simulink model "TwoLevel_ThreePhase_PWM_2017b"  (R2017b)
settings: Solver=VariableStepAuto  StartTime=0.0  StopTime=0.1  RelTol=1e-3
StopFcn:
  | Vabc=out.Vabcn;
  | Vab=out.Vab;
  | Iabc=out.Iabcn;
libraries: powerlib x12, simulink x4
settings Model: Creator=defus  LastModifiedBy=Mehdi
settings DataIOCC: ReturnWorkspaceOutputs=on
settings DebuggingCC: UnconnectedInputMsg=none  UnconnectedOutputMsg=none  UnconnectedLineMsg=none
settings ModelReferenceCC: EnableRefExpFcnMdlSchedulingChecks=off
settings SFSimCC: SimUseLocalCustomCode=on
settings RTWCC: Description=Generic Real-Time Target  RTWUseLocalCustomCode=on
settings CodeAppCC: StateflowObjectComments=on
settings SimscapeCC: SimscapeNormalizeSystem=off

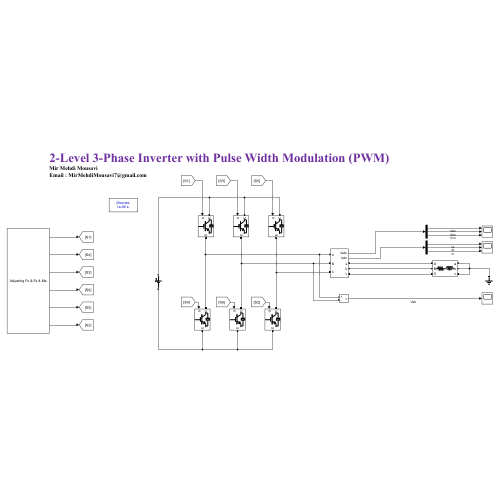
[thumbnail: Simulink's stored preview of the top-level diagram]
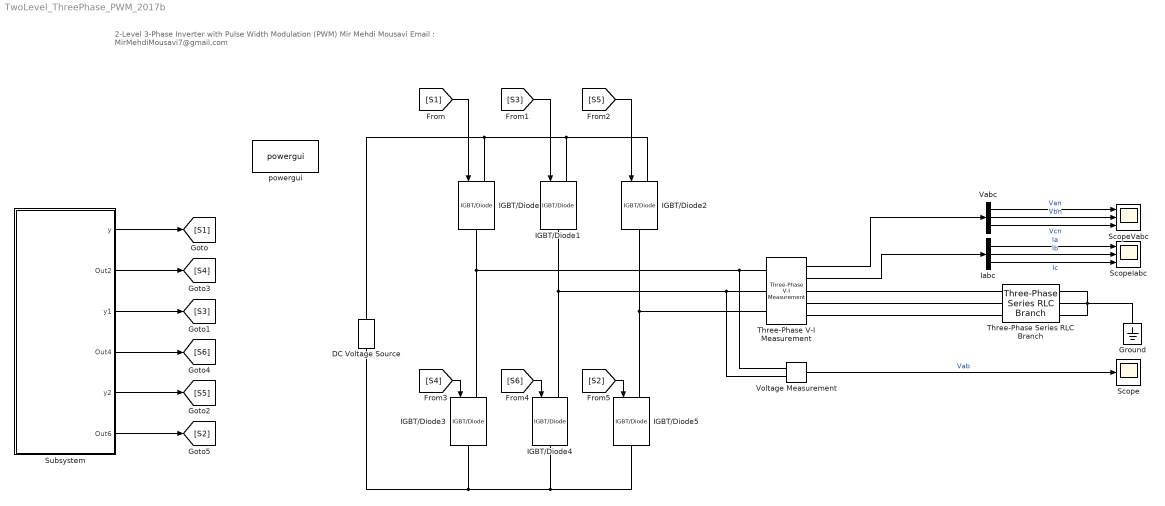
== system TwoLevel_ThreePhase_PWM_2017b ==
  note: 2-Level 3-Phase Inverter with Pulse Width Modulation (PWM)
      | Mir Mehdi Mousavi
      | Email : MirMehdiMousavi7@gmail.com
  DC Voltage Source : powerlib/Electrical Sources/DC Voltage Source  Amplitude=400  Measurements=None
  Ground : powerlib/Elements/Ground  LConnTagsString=a
  IGBT/Diode{,1..5} (6 alike) : powerlib/Power Electronics/IGBT//Diode  Ron=1e-3  Rs=1e5  Cs=inf  Measurements=off
  Iabc : Demux  Outputs=3
  Scope : Scope
  ScopeIabc : Scope  NumInputPorts=3
  ScopeVabc : Scope  NumInputPorts=3
  Subsystem : Subsystem  mask{fo=50, fs=1750, ma=1}
      mask prompts: fo "Output Frequency (Hz)"; fs "Sitching Frequency (Hz)"; ma "Index Modulation"
      mask Display: fprintf('Adjusting Fo & Fs & Ma')
  Three-Phase Series RLC Branch : powerlib/Elements/Three-Phase Series RLC Branch  LConnTagsString=A|B|C  RConnTagsString=A|B|C  BranchType=RL  Resistance=3  Inductance=1.5e-2  Capacitance=1e-6  Measurements=None
  Three-Phase V-I Measurement : powerlib/Measurements/Three-Phase V-I Measurement  VoltageMeasurement=phase-to-ground  SetLabelV=off  LabelV=Vabc  Vpu=off  VpuLL=off  CurrentMeasurement=yes  SetLabelI=off  LabelI=Iabc  Ipu=off  Pbase=100e6  Vbase=500e3  OutputType=Complex  PhasorSimulation=off  PSBequivalent=0
  Vabc : Demux  Outputs=3
  Voltage Measurement : powerlib/Measurements/Voltage Measurement  PhasorSimulation=off  OutputType=Complex  PSBequivalent=0
  powergui : powerlib/powergui  Priority=1  SimulationMode=Discrete  SampleTime=1e-6  frequency=60  Iterations=50  frequencyindice=0  Pbase=100e6  ErrMax=1e-4  UnitsV=kV  UnitsW=MW  buscounter=0  FunctionMessages=off  echomessages=off  EnableUseOfTLC=off  CurrentSourceSwitches=off  DisableSnubberDevices=off  DisableRonSwitches=off  DisableVfSwitches=off  DisplayEquations=off  AutomaticDiscreteSolvers=off  SolverType=Tustin/Backward Euler (TBE)  Interpol=off  ExternalGateDelay=off  methode=off  Ts=100  x0status=blocks  SPID=on  SwTol=0  HookPort=off  NonlinearTolerance=1e-4  nMaxIteration=100  ContinueOnMaxIteration=off  RestoreLinks=warning  ResistiveCurrentMeasurement=off  Frange=[0:2:500]  Ylog=off  Xlog=on  ShowGrid=off  save=off  variable=ZData  structure=0  ZoomFFT=off  StartTime=0.0  cycles=1  DisplayStyle=1  fundamental=60  FreqAxis=off  MaxFrequency=1000  frequencyindicesteady=1  RmsSteady=1  display=off
  wires:
  [S1] -> IGBT/Diode/1
  [S3] -> IGBT/Diode1/1
  [S5] -> IGBT/Diode2/1
  [S4] -> IGBT/Diode3/1
  [S2] -> IGBT/Diode5/1
  [S6] -> IGBT/Diode4/1
  Subsystem/1(y) -> [S1]
  Subsystem/2(Out2) -> [S4]
  Subsystem/3(y1) -> [S3]
  Subsystem/4(Out4) -> [S6]
  Subsystem/5(y2) -> [S5]
  Subsystem/6(Out6) -> [S2]
  Vabc/2 -> ScopeVabc/2  "Vbn"
  Three-Phase V-I Measurement/1 -> Vabc/1
  Three-Phase V-I Measurement/2 -> Iabc/1
  Voltage Measurement/1 -> Scope/1  "Vab"
  Iabc/2 -> ScopeIabc/2  "Ib"
  Vabc/1 -> ScopeVabc/1  "Van"
  Vabc/3 -> ScopeVabc/3  "Vcn"
  Iabc/1 -> ScopeIabc/1  "Ia"
  Iabc/3 -> ScopeIabc/3  "Ic"
  connections:
  IGBT/Diode/LConn1 -- DC Voltage Source/RConn1 -- IGBT/Diode2/LConn1 -- IGBT/Diode1/LConn1
  DC Voltage Source/LConn1 -- IGBT/Diode3/RConn1 -- IGBT/Diode5/RConn1 -- IGBT/Diode4/RConn1
  IGBT/Diode/RConn1 -- Voltage Measurement/LConn1 -- Three-Phase V-I Measurement/LConn1 -- IGBT/Diode3/LConn1
  IGBT/Diode1/RConn1 -- Voltage Measurement/LConn2 -- Three-Phase V-I Measurement/LConn2 -- IGBT/Diode4/LConn1
  IGBT/Diode2/RConn1 -- IGBT/Diode5/LConn1 -- Three-Phase V-I Measurement/LConn3
  Three-Phase Series RLC Branch/RConn3 -- Three-Phase Series RLC Branch/RConn2 -- Ground/LConn1 -- Three-Phase Series RLC Branch/RConn1
  Three-Phase V-I Measurement/RConn2 -- Three-Phase Series RLC Branch/LConn2
  Three-Phase V-I Measurement/RConn1 -- Three-Phase Series RLC Branch/LConn1
  Three-Phase V-I Measurement/RConn3 -- Three-Phase Series RLC Branch/LConn3

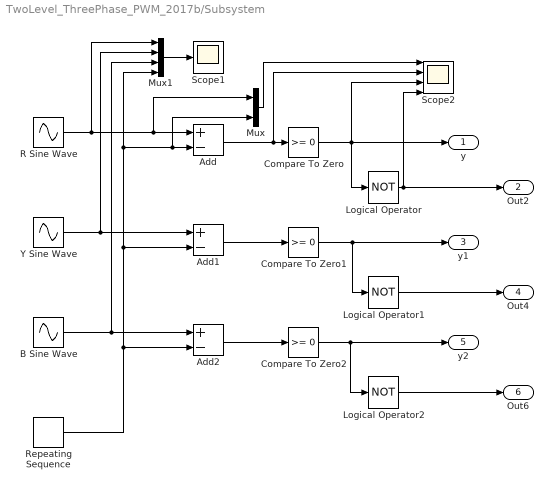
== system TwoLevel_ThreePhase_PWM_2017b/Subsystem ==
  Add : Sum  Inputs=+-
  Add1 : Sum  Inputs=+-
  Add2 : Sum  Inputs=+-
  B Sine Wave : Sin  Amplitude=ma  Frequency=2*pi*fo  Phase=-2*pi/3  SampleTime=1e-06
  Compare To Zero : simulink/Logic and Bit Operations/Compare To Zero  relop=>=  OutDataTypeStr=boolean
  Compare To Zero1 : simulink/Logic and Bit Operations/Compare To Zero  relop=>=  OutDataTypeStr=boolean
  Compare To Zero2 : simulink/Logic and Bit Operations/Compare To Zero  relop=>=  OutDataTypeStr=boolean
  Logical Operator : Logic  Operator=NOT  AllPortsSameDT=off  OutDataTypeStr=boolean
  Logical Operator1 : Logic  Operator=NOT  AllPortsSameDT=off  OutDataTypeStr=boolean
  Logical Operator2 : Logic  Operator=NOT  AllPortsSameDT=off  OutDataTypeStr=boolean
  Mux : Mux  Inputs=2
  Mux1 : Mux
  R Sine Wave : Sin  Amplitude=ma  Frequency=2*pi*fo  SampleTime=1e-06
  Repeating Sequence : simulink/Sources/Repeating Sequence  rep_seq_t=[0 1 2 3 4]*[1/(4*fs)]  rep_seq_y=[0 1 0 -1 0]
  Scope1 : Scope
  Scope2 : Scope  NumInputPorts=4
  Y Sine Wave : Sin  Amplitude=ma  Frequency=2*pi*fo  Phase=2*pi/3  SampleTime=1e-06
  y : Outport
  Out2 : Outport  Port=2
  y1 : Outport  Port=3
  Out4 : Outport  Port=4
  y2 : Outport  Port=5
  Out6 : Outport  Port=6
  wires:
  Add2/1 -> Compare To Zero2/1
  Repeating Sequence/1 -> Mux1/4, Mux/2, Add/2, Add1/2, Add2/2
  Add1/1 -> Compare To Zero1/1
  Compare To Zero/1 -> y/1, Scope2/3, Logical Operator/1
  B Sine Wave/1 -> Mux1/3, Add2/1
  Compare To Zero1/1 -> y1/1, Logical Operator1/1
  R Sine Wave/1 -> Mux1/1, Add/1, Mux/1
  Compare To Zero2/1 -> y2/1, Logical Operator2/1
  Mux1/1 -> Scope1/1
  Logical Operator/1 -> Out2/1, Scope2/4
  Add/1 -> Scope2/2, Compare To Zero/1
  Y Sine Wave/1 -> Add1/1, Mux1/2
  Logical Operator1/1 -> Out4/1
  Mux/1 -> Scope2/1
  Logical Operator2/1 -> Out6/1
